simulink model "vehicle_model_controller_ref"  (R2020b)
settings: Solver=VariableStepAuto  StartTime=0.0  StopTime=180  FixedStep=0.001  RelTol=1e-3
model workspace (MAT data in the model file):
  understeer_gradient = 0.05
undefined symbols (not defined in the file or in its folder): front_forces, rear_forces
libraries: fl_lib x24, nesl_utility x20, sdl_lib x8, autolibmappedmotor x4, vehdynlibsteering x1, pid_lib x1, autolibshared x1, autolibdatasheetbattery x1
(part 4 of 4)

== matlab function vehicle_model_controller_ref/Driver Input Logic/Torque Vectoring Controller/LP model ==
  data: s input; T_x_ij output; l input; PID input; delta input; driver_input input; F_x_ij_max input; F_y_ij input; sum_torque output; yaw_rate_y output
function [T_x_ij, sum_torque, yaw_rate_y]= LP(s, l, PID, delta, driver_input, F_x_ij_max, F_y_ij)
%% Two-track model equation of motion
% Developers:    David Farell
%                Elliot Stockwell
% Developed for: Purdue Electric Racing
% Date:          04/24/2021
%
% Definitions:
% s:        half track width vector                 [m]
% l:        wheelbase vector                        [m]
% delta:    steering angle vector                   [deg]
% PID:      efficacy of LP based on error           [N]
% F_x_ij_max:   maximum longitudinal tire force vector          [N]
% F_y_ij: Lateral force on the car                              [N]
% driver_input: maximum total force motors can output           [N]

%% Constants
J_z = 4000;     % Inertia moment                            [kg * m^2]
s_f = s(1);     % half track width front                    [m]
s_r = s(2);     % half track width rear                     [m]
l_f = l(1);     % wheelbase front                           [m]
l_r = l(2);     % wheelbase rear                            [m]
R = 0.3;        % radius                                    [m]
GR_f = (37/24) * (84/23) + 1;   % front gear ratio          [unitless]
GR_r = (40/21) * (84/23) + 1;   % rear gear ratio           [unitless]

%% Defining EOM vector K_1
% x_1 component of EOM vector in K_1
x_1 = (s_f * cos(delta(1))) + (l_f * sin(delta(1)));    
% x_2 component of EOM vector in K_1
x_2 = (-1 * s_f * cos(delta(2))) + (l_f * sin(delta(2)));     
% x_3 component of EOM vector in K_1
x_3 = s_r;     
% x_4 component of EOM vector in K_1
x_4 = -s_r; 
% EOM vector in K_1
x = [x_1; x_2; x_3; x_4]; 

% K_1 vector of vehicle constants and parameters
K_1 = (1 / J_z) * x; 

%% Defining EOM linear combination K_2
% y_1 component of EOM linear combination in K_2
y_1 = (-1 * s_f * sin(delta(1))) + (l_f * cos(delta(1)));    
% y_2 component of EOM linear combination in K_2
y_2 = (s_f * sin(delta(2))) + (l_f * cos(delta(2)));
% y_3 component of EOM linear combination in K_2
y_3 = -l_r;
% y_4 component of EOM vector in K_2
y_4 = -l_r;
% EOM vector in K_2
y = [y_1; y_2; y_3; y_4]; 

% K_2 vector of vehicle constants and parameters and lateral wheel forces
K_2 = (1 / J_z) * y;
yaw_rate_y = sum(K_2 .* F_y_ij);


%% Linear Programming Model
% The output of the linear programming model is a variable F_x_ij_mod

% Define objective function and optimization variables
% C1, C2, C3, C4, the force-to-torque conversion for each wheel
f = [-GR_f/GR_r, -GR_f/GR_r, -1, -1];
 
% generate the objective function
objfun = @(x) sum(x.*f);

% the start point for the algorithm
x0 = [10, 10, 10, 10];

% inequality vector, less than side
A = [1, 1, 1, 1; -1, -1, 1, 1;];

% inequality vector, greater than side
b = [driver_input, driver_input];

% equality vector, the side with objective variables
Aeq = K_1' .* f;

% equality vector, the side without objective variables
beq = -yaw_rate_y + PID;

% lower boundary for each objective variable
lb = [-10, -10, -10, -10];

% upper boundary for each objective variable
ub = [10, 10, 10, 10];

% set which algorithm the optimization function is going to use
options = optimoptions('fmincon','Algorithm','sqp');

% find the optimal solution
[F_x_ij] = fmincon(objfun,x0,A,b,Aeq,beq,lb,ub,[],options);

% convert force to torque
T_x_ij = (F_x_ij .* R)';
sum_torque = sum(F_x_ij);

== matlab function vehicle_model_controller_ref/Driver Input Logic/Torque Vectoring Controller/Reference yaw rate processor/Desired yaw rate ==
  data: steering_angle input; K_u input; l input; x_dot input; y_dot input; psi_1_des output
function psi_1_des = des_yaw_rate(steering_angle, K_u, l, x_dot, y_dot)
%% Desired yaw rate
% Developers:    David Farell
%                Elliot Stockwell
% Developed for: Purdue Electric Racing
% Date:          04/24/2021
%
% Definitions:
% x_dot:    longitudinal velocity at CoG            [m * s^-1]
% y_dot:    lateral velocity at CoG                 [m * s^-1]
% l:        wheelbase vector                        [m]
% K_u:      under-steer gradient                    [unitless]
% delta:    steering angle                          [deg]

%% Constants
v_cog = sqrt(x_dot^2 + y_dot^2); % speed at CoG            [m * s^-1]
l_f = l(1);      % wheelbase front                         [m]
l_r = l(2);      % wheelbase rear                          [m]

%% Desired yaw rate
psi_1_des = (v_cog * abs(steering_angle)) / ((l_f + l_r) + (K_u * v_cog ^ 2));
% calculates desired yaw rate based on the equations given in the TV paper
% by Anton Stoop

== matlab function vehicle_model_controller_ref/Driver Input Logic/Torque Vectoring Controller/Reference yaw rate processor/Maximum yaw rate ==
  data: x_dot input; y_dot input; psi_1_max output; mu_max input
function psi_1_max = max_yaw_rate(x_dot, y_dot, mu_max)
%% Maximum yaw rate
% Developers:    David Farell
%                Elliot Stockwell
% Developed for: Purdue Electric Racing
% Date:          04/24/2021
%
% Definitions:
% x_dot:    longitudinal velocity at CoG            [m * s^-1]
% y_dot:    lateral velocity at CoG                 [m * s^-1]
% mu_max:   maximum friction coefficient            [unitless]

%% Constants
g = 9.806;       % acceleration due to gravity             [m / s^-2]

%% Calculations
v_cog = sqrt(x_dot^2 + y_dot^2); % speed at CoG            [m * s^-1]
mu_max = max(max(mu_max)); % maximum overall friction coefficient 

%% Maximum yaw rate
psi_1_max = (mu_max * g) / (v_cog + 0.05);

== matlab function vehicle_model_controller_ref/Driver Input Logic/Torque Vectoring Controller/Maximum longitudinal force, no slip ==
  data: mu_max input; delta input; alpha input; F_z_ij input; F_x_ij input; F_x_ij_max output
function F_x_ij_max = LP_F_x_max_noslip(mu_max, delta, alpha, ...
      F_z_ij, F_x_ij)
%% Linear programming max longitudinal force before loss of traction
% Developers:    David Farell
%                Elliot Stockwell
% Developed for: Purdue Electric Racing
% Date:          04/24/2021
%
% Definitions:
% F_x_ij:   Tire lateral force vector               [N]
% F_z_ij:   Tire loading vector                     [N]
% mu_max:   Maximum friction coefficient            [m/s]
% alpha:    Slip angle vector                       [rad]
% delta:    Steering angle                          [rad]
% req_f:    Driver requested force                  [N]

%% Constants
delta_o = [delta(1); delta(2); 0; 0];
mu_max = [mu_max(1:2), mu_max(3:4)]';

%% Maximum longitudinal forces in the direction of wheel velocity
F_wl = sqrt((mu_max .* F_z_ij).^2 + F_x_ij.^2);

%% Maximum longitudinal and lateral forces in the wheel coordinates
F_l = F_wl .* cos(alpha) + F_x_ij .* sin(alpha);
F_s = F_x_ij .* cos(alpha) - F_wl .* sin(alpha);

% Maximum longitudinal forces in undercarriage coordinates
F_x_ij_max = F_l .* cos(delta_o) - F_s .* sin(delta_o);

== matlab function vehicle_model_controller_ref/Driver Input Logic/Torque Vectoring Controller/MATLAB Function ==
  data: delta input; y_dot input; x_dot input; r input; w input; alpha output; s input
function alpha = slip_angle(delta, y_dot, x_dot, r, w, s)
%% Front and rear slip angle
% Developers:    David Farell
%                Elliot Stockwell
% Developed for: Purdue Electric Racing
% Date:          04/27/2021
%
% Definitions:
% y_dot:    Vehicle CoG lateral velocity            [m/s]
% x_dot:    Vehicle CoG longitudinal velocity       [m/s]    
% a:        Distance from front wheel axle to CoG   [m]
% b:        Distance from rear wheel axle to CoG    [m]
% r:        Vehicle angular velocity                [rad/s]
% w:        Wheelbase vector                        [m]
% delta:    Steering angle vector                   [rad]

%% Constants
a = s(1);
b = s(2);
w_f = w(1);
w_r = w(2);
delta_fl = delta(1);
delta_fr = delta(2);
delta_rl = 0;
delta_rr = 0;

%% Front left slip angle
alpha_fl = atan((y_dot + a * r) / (x_dot + r * w_f / 2)) - delta_fl;

%% Front right slip angle
alpha_fr = atan((y_dot + a * r) / (x_dot - r * w_f / 2)) - delta_fr;

%% Rear left slip angle
alpha_rl = atan((y_dot - b * r) / (x_dot + r * w_r / 2)) - delta_rl;

%% Rear right slip angle
alpha_rr = atan((y_dot - b * r) / (x_dot - r * w_r / 2)) - delta_rr;


%% Slip angle vector
alpha = [alpha_fl; alpha_fr; alpha_rl; alpha_rr];

== matlab function vehicle_model_controller_ref/Driver Input Logic/Braking Controller/MATLAB Function ==
  data: driver_input input; T_x_ij output
function T_x_ij = split_braking_torque(driver_input)
%% Regenerative Braking Force Split
% Developers:    Demetrius Gulewicz
% Developed for: Purdue Electric Racing
% Date:          09/01/2021
%
% Definitions:
% driver_input:   sum of forces requested by driver to the 4 motors   [N]
%% Constants
R = 0.3;        % wheel radius                              [m]


%% Calculation
driver_torque = (driver_input * R)/ 4;


T_x_ij = [driver_torque; driver_torque; driver_torque; driver_torque];

== matlab function vehicle_model_controller_ref/Driver Input Logic/Torque Vectoring Controller/MATLAB Function1 ==
  data: F_x_ij_abs input; F_y_ij_abs input; delta input; F_y_ij output
function F_y_ij = Calculate_F_y_ij(F_x_ij_abs, F_y_ij_abs, delta)

F_y_ij = [0; 0; 0; 0];

F_y_ij(1) = (sin(delta(1)) * F_x_ij_abs(1)) + (cos(delta(1)) * F_y_ij_abs(1));

F_y_ij(2) = (sin(delta(2)) * F_x_ij_abs(2)) + (cos(delta(2)) * F_y_ij_abs(2));

F_y_ij(3) = F_y_ij_abs(3);

F_y_ij(4) = F_y_ij_abs(4);
